simulink library "SHLI_lib"  (Simulink 7.5)
settings: Solver=ode45  StartTime=0.0  StopTime=10.0  RelTol=1e-3
values from neighbouring files (symbols this model uses):
  pSHLI_bool_EparkCheckEnbl = Simulink.Parameter    [SHLI_FAW_par.m]
  pSHLI_bool_EparkStEnbl = Simulink.Parameter    [SHLI_FAW_par.m]
  pSHLI_bool_SBWSafeBtnDisEnbl = Simulink.Parameter    [SHLI_FAW_par.m]
  pSHLI_st_EparkStUnPark = Simulink.Parameter    [SHLI_FAW_par.m]
undefined symbols (not defined in the file or in its folder): EparkModTyp, OperProfTyp, p_bool_False_M, p_bool_True_M, PrkgLockBtnTyp, PrkgLockStsTyp, ShiftLvrPosnTipTyp
libraries: BaseOperationLib_Browser x29, PES_CZ_FAW x3, simulink x1
settings Model: Creator=wuaibin  LastModifiedBy=wuaibin

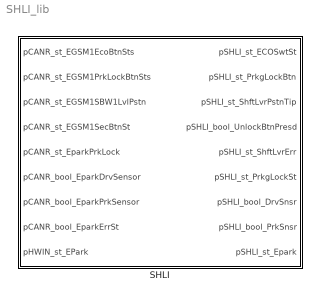
== system SHLI_lib ==
  SHLI : Subsystem  TreatAsAtomicUnit=on

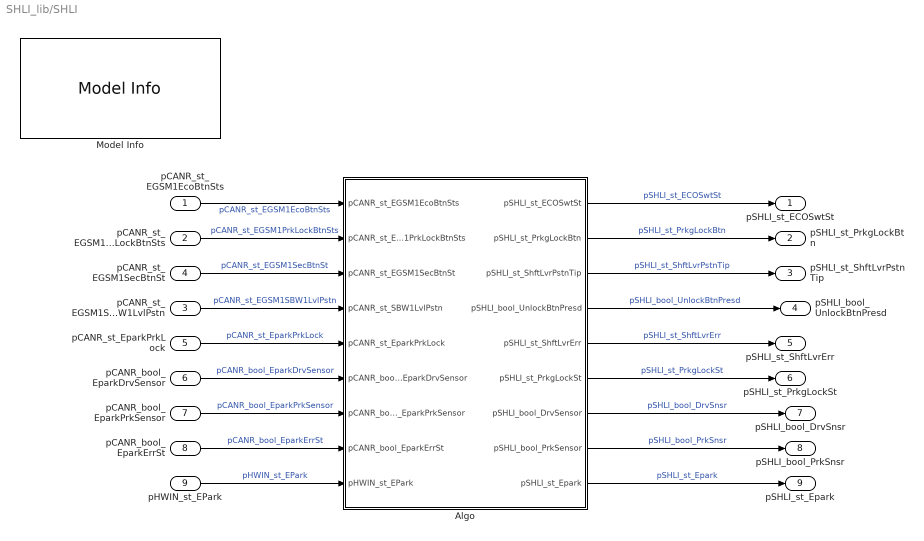
== system SHLI_lib/SHLI ==
  pCANR_st_EGSM1EcoBtnSts : Inport  OutDataType=fixdt(1, 16)  OutScaling=2^0
  pCANR_st_EGSM1PrkLockBtnSts : Inport  Port=2  OutDataType=fixdt(1, 16)  OutScaling=2^0
  pCANR_st_EGSM1SBW1LvlPstn : Inport  Port=3  OutDataType=fixdt(1, 16)  OutScaling=2^0
  pCANR_st_EGSM1SecBtnSt : Inport  Port=4  OutDataType=fixdt(1, 16)  OutScaling=2^0
  pCANR_st_EparkPrkLock : Inport  Port=5  OutDataType=fixdt(1, 16)  OutScaling=2^0
  pCANR_bool_EparkDrvSensor : Inport  Port=6  OutDataType=fixdt(1, 16)  OutScaling=2^0
  pCANR_bool_EparkPrkSensor : Inport  Port=7  OutDataType=fixdt(1, 16)  OutScaling=2^0
  pCANR_bool_EparkErrSt : Inport  Port=8  OutDataType=fixdt(1, 16)  OutScaling=2^0
  pHWIN_st_EPark : Inport  Port=9  OutDataType=fixdt(1, 16)  OutScaling=2^0
  Algo : Subsystem
  Model Info : simulink/Model-Wide Utilities/Model Info  SystemSampleTime=-1  InitialBlockCM=None  BlockCM=None  Frame=on  DisplayStringWithTags=Model Info\nCreated: %<Created>\nCreator: wuaibin  HorizontalTextAlignment=Center  LeftAlignmentValue=0.5  SourceBlockDiagram=HQEV_HCU  TagMaxNumber=20
  pSHLI_st_ECOSwtSt : Outport  OutDataType=fixdt(1, 16)  OutScaling=2^0
  pSHLI_st_PrkgLockBtn : Outport  Port=2  OutDataType=fixdt(1, 16)  OutScaling=2^0
  pSHLI_st_ShftLvrPstnTip : Outport  Port=3  OutDataType=fixdt(1, 16)  OutScaling=2^0
  pSHLI_bool_UnlockBtnPresd : Outport  Port=4  OutDataType=fixdt(1, 16)  OutScaling=2^0
  pSHLI_st_ShftLvrErr : Outport  Port=5  OutDataType=fixdt(1, 16)  OutScaling=2^0
  pSHLI_st_PrkgLockSt : Outport  Port=6  OutDataType=fixdt(1, 16)  OutScaling=2^0
  pSHLI_bool_DrvSnsr : Outport  Port=7  OutDataType=fixdt(1, 16)  OutScaling=2^0
  pSHLI_bool_PrkSnsr : Outport  Port=8  OutDataType=fixdt(1, 16)  OutScaling=2^0
  pSHLI_st_Epark : Outport  Port=9  OutDataType=fixdt(1, 16)  OutScaling=2^0
  wires:
  pCANR_st_EGSM1SBW1LvlPstn/1 -> Algo/4(pCANR_st_SBW1LvlPstn)  "pCANR_st_EGSM1SBW1LvlPstn"
  Algo/2(pSHLI_st_PrkgLockBtn) -> pSHLI_st_PrkgLockBtn/1  "pSHLI_st_PrkgLockBtn"
  Algo/6(pSHLI_st_PrkgLockSt) -> pSHLI_st_PrkgLockSt/1  "pSHLI_st_PrkgLockSt"
  pCANR_st_EGSM1PrkLockBtnSts/1 -> Algo/2(pCANR_st_EGSM1PrkLockBtnSts)  "pCANR_st_EGSM1PrkLockBtnSts"
  Algo/5(pSHLI_st_ShftLvrErr) -> pSHLI_st_ShftLvrErr/1  "pSHLI_st_ShftLvrErr"
  Algo/3(pSHLI_st_ShftLvrPstnTip) -> pSHLI_st_ShftLvrPstnTip/1  "pSHLI_st_ShftLvrPstnTip"
  pCANR_st_EGSM1EcoBtnSts/1 -> Algo/1(pCANR_st_EGSM1EcoBtnSts)  "pCANR_st_EGSM1EcoBtnSts"
  Algo/1(pSHLI_st_ECOSwtSt) -> pSHLI_st_ECOSwtSt/1  "pSHLI_st_ECOSwtSt"
  Algo/8(pSHLI_bool_PrkSensor) -> pSHLI_bool_PrkSnsr/1  "pSHLI_bool_PrkSnsr"
  pCANR_bool_EparkErrSt/1 -> Algo/8(pCANR_bool_EparkErrSt)  "pCANR_bool_EparkErrSt"
  pCANR_bool_EparkDrvSensor/1 -> Algo/6(pCANR_bool_EparkDrvSensor)  "pCANR_bool_EparkDrvSensor"
  pCANR_bool_EparkPrkSensor/1 -> Algo/7(pCANR_bool_EparkPrkSensor)  "pCANR_bool_EparkPrkSensor"
  pCANR_st_EparkPrkLock/1 -> Algo/5(pCANR_st_EparkPrkLock)  "pCANR_st_EparkPrkLock"
  pCANR_st_EGSM1SecBtnSt/1 -> Algo/3(pCANR_st_EGSM1SecBtnSt)  "pCANR_st_EGSM1SecBtnSt"
  pHWIN_st_EPark/1 -> Algo/9(pHWIN_st_EPark)  "pHWIN_st_EPark"
  Algo/9(pSHLI_st_Epark) -> pSHLI_st_Epark/1  "pSHLI_st_Epark"
  Algo/4(pSHLI_bool_UnlockBtnPresd) -> pSHLI_bool_UnlockBtnPresd/1  "pSHLI_bool_UnlockBtnPresd"
  Algo/7(pSHLI_bool_DrvSensor) -> pSHLI_bool_DrvSnsr/1  "pSHLI_bool_DrvSnsr"

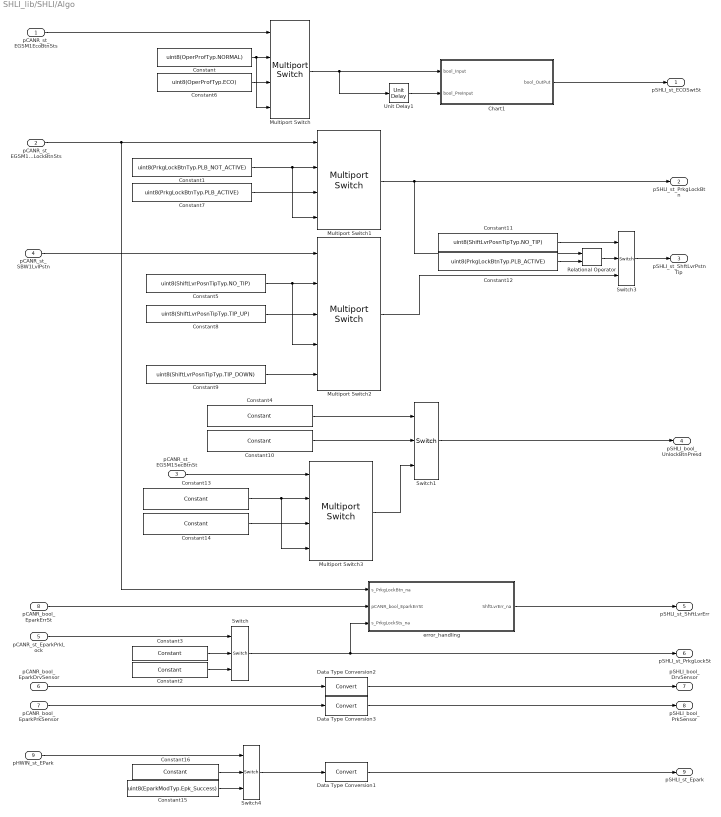
== system SHLI_lib/SHLI/Algo ==
  pCANR_st_EGSM1EcoBtnSts : Inport  OutDataType=fixdt(1, 16)  OutScaling=2^0
  pCANR_st_EGSM1PrkLockBtnSts : Inport  Port=2  OutDataType=fixdt(1, 16)  OutScaling=2^0
  pCANR_st_EGSM1SecBtnSt : Inport  Port=3  OutDataType=fixdt(1, 16)  OutScaling=2^0
  pCANR_st_SBW1LvlPstn : Inport  Port=4  OutDataType=fixdt(1, 16)  OutScaling=2^0
  pCANR_st_EparkPrkLock : Inport  Port=5  OutDataType=fixdt(1, 16)  OutScaling=2^0
  pCANR_bool_EparkDrvSensor : Inport  Port=6  OutDataType=fixdt(1, 16)  OutScaling=2^0
  pCANR_bool_EparkPrkSensor : Inport  Port=7  OutDataType=fixdt(1, 16)  OutScaling=2^0
  pCANR_bool_EparkErrSt : Inport  Port=8  OutDataType=fixdt(1, 16)  OutScaling=2^0
  pHWIN_st_EPark : Inport  Port=9  OutDataType=fixdt(1, 16)  OutScaling=2^0
  Chart1 : Stateflow chart  TreatAsAtomicUnit=on
  Constant : Constant  Value=uint8(OperProfTyp.NORMAL)  OutDataType=fixdt(1, 16)  OutScaling=2^0
      mask Display: patch([0 1 1 1 .75], [1 1 0 .75 1], [0 1 0]);
  Constant1 : Constant  Value=uint8(PrkgLockBtnTyp.PLB_NOT_ACTIVE)  OutDataType=fixdt(1, 16)  OutScaling=2^0
      mask Display: patch([0 1 1 1 .75], [1 1 0 .75 1], [0 1 0]);
  Constant10 : BaseOperationLib_Browser/Sources&Sinks/Constant  Value=pSHLI_bool_SBWSafeBtnDisEnbl  OutMin=[]  OutMax=[]  OutDataType=fixdt(1, 16)  ConRadixGroup=Use specified scaling  OutScaling=2^0  OutDataTypeStr=Inherit: Inherit from 'Constant value'
  Constant11 : Constant  Value=uint8(ShiftLvrPosnTipTyp.NO_TIP)  OutDataType=fixdt(1, 16)  OutScaling=2^0
      mask Display: patch([0 1 1 1 .75], [1 1 0 .75 1], [0 1 0]);
  Constant12 : Constant  Value=uint8(PrkgLockBtnTyp.PLB_ACTIVE)  OutDataType=fixdt(1, 16)  OutScaling=2^0
      mask Display: patch([0 1 1 1 .75], [1 1 0 .75 1], [0 1 0]);
  Constant13 : BaseOperationLib_Browser/Sources&Sinks/Constant  Value=p_bool_False_M  OutMin=[]  OutMax=[]  OutDataType=fixdt(1, 16)  ConRadixGroup=Use specified scaling  OutScaling=2^0  OutDataTypeStr=Inherit: Inherit from 'Constant value'
  Constant14 : BaseOperationLib_Browser/Sources&Sinks/Constant  Value=p_bool_True_M  OutMin=[]  OutMax=[]  OutDataType=fixdt(1, 16)  ConRadixGroup=Use specified scaling  OutScaling=2^0  OutDataTypeStr=Inherit: Inherit from 'Constant value'
  Constant15 : Constant  Value=uint8(EparkModTyp.Epk_Success)  OutDataTypeMode=uint8  OutDataType=fixdt(1, 16)  OutScaling=2^0  OutDataTypeStr=uint8
  Constant16 : BaseOperationLib_Browser/Sources&Sinks/Constant  Value=pSHLI_bool_EparkCheckEnbl  OutMin=[]  OutMax=[]  OutDataType=fixdt(1, 16)  ConRadixGroup=Use specified scaling  OutScaling=2^0  OutDataTypeStr=Inherit: Inherit from 'Constant value'
  Constant2 : BaseOperationLib_Browser/Sources&Sinks/Constant  Value=pSHLI_st_EparkStUnPark  OutMin=[]  OutMax=[]  OutDataType=fixdt(1, 16)  ConRadixGroup=Use specified scaling  OutScaling=2^0  OutDataTypeStr=Inherit: Inherit from 'Constant value'
  Constant3 : BaseOperationLib_Browser/Sources&Sinks/Constant  Value=pSHLI_bool_EparkStEnbl  OutMin=[]  OutMax=[]  OutDataType=fixdt(1, 16)  ConRadixGroup=Use specified scaling  OutScaling=2^0  OutDataTypeStr=Inherit: Inherit from 'Constant value'
  Constant4 : BaseOperationLib_Browser/Sources&Sinks/Constant  Value=p_bool_True_M  OutMin=[]  OutMax=[]  OutDataType=fixdt(1, 16)  ConRadixGroup=Use specified scaling  OutScaling=2^0  OutDataTypeStr=Inherit: Inherit from 'Constant value'
  Constant5 : Constant  Value=uint8(ShiftLvrPosnTipTyp.NO_TIP)  OutDataType=fixdt(1, 16)  OutScaling=2^0
      mask Display: patch([0 1 1 1 .75], [1 1 0 .75 1], [0 1 0]);
  Constant6 : Constant  Value=uint8(OperProfTyp.ECO)  OutDataType=fixdt(1, 16)  OutScaling=2^0
      mask Display: patch([0 1 1 1 .75], [1 1 0 .75 1], [0 1 0]);
  Constant7 : Constant  Value=uint8(PrkgLockBtnTyp.PLB_ACTIVE)  OutDataType=fixdt(1, 16)  OutScaling=2^0
      mask Display: patch([0 1 1 1 .75], [1 1 0 .75 1], [0 1 0]);
  Constant8 : Constant  Value=uint8(ShiftLvrPosnTipTyp.TIP_UP)  OutDataType=fixdt(1, 16)  OutScaling=2^0
      mask Display: patch([0 1 1 1 .75], [1 1 0 .75 1], [0 1 0]);
  Constant9 : Constant  Value=uint8(ShiftLvrPosnTipTyp.TIP_DOWN)  OutDataType=fixdt(1, 16)  OutScaling=2^0
      mask Display: patch([0 1 1 1 .75], [1 1 0 .75 1], [0 1 0]);
  Data Type Conversion1 : DataTypeConversion  OutDataType=fixdt(1, 16)  OutScaling=2^0
  Data Type Conversion2 : DataTypeConversion  OutDataType=fixdt(1, 16)  OutScaling=2^0
  Data Type Conversion3 : DataTypeConversion  OutDataType=fixdt(1, 16)  OutScaling=2^0
  Multiport Switch : BaseOperationLib_Browser/Signal Routing Changed/Multiport Switch  DataPortOrder=Specify indices  Inputs=3  DataPortIndices={uint8(EcoBtnStsTyp.ECO_OFF),uint8(EcoBtnStsTyp.ECO_ON),uint8(EcoBtnStsTyp.ECO_ERROR)}  zeroidx=off  InputSameDT=on  OutMin=[]  OutMax=[]  OutDataType=fixdt(1, 16)  OutScaling=2^0  SaturateOnIntegerOverflow=on
  Multiport Switch1 : BaseOperationLib_Browser/Signal Routing Changed/Multiport Switch  DataPortOrder=Specify indices  Inputs=3  DataPortIndices={uint8(PrkgLockBtnTyp.PLB_NOT_ACTIVE),uint8(PrkgLockBtnTyp.PLB_ACTIVE),uint8(PrkgLockBtnTyp.PLB_ERROR)}  zeroidx=off  InputSameDT=on  OutMin=[]  OutMax=[]  OutDataType=fixdt(1, 16)  OutScaling=2^0  SaturateOnIntegerOverflow=on
  Multiport Switch2 : BaseOperationLib_Browser/Signal Routing Changed/Multiport Switch  DataPortOrder=Specify indices  Inputs=4  DataPortIndices={uint8(FAWShiftLvrPosnTipTyp.FAWTIP_NO_TIP), uint8(FAWShiftLvrPosnTipTyp.FAWTIP_UP), uint8(FAWShiftLvrPosnTipTyp.FAWTIP_DOWN), uint8(FAWShiftLvrPosnTipTyp.FAWTIP_ERROR)}  zeroidx=off  InputSameDT=on  OutMin=[]  OutMax=[]  OutDataType=fixdt(1, 16)  OutScaling=2^0  SaturateOnIntegerOverflow=on
  Multiport Switch3 : BaseOperationLib_Browser/Signal Routing Changed/Multiport Switch  DataPortOrder=Specify indices  Inputs=3  DataPortIndices={uint8(PrkgLockBtnTyp.PLB_NOT_ACTIVE),uint8(PrkgLockBtnTyp.PLB_ACTIVE),uint8(PrkgLockBtnTyp.PLB_ERROR)}  zeroidx=off  InputSameDT=on  OutMin=[]  OutMax=[]  OutDataType=fixdt(1, 16)  OutScaling=2^0  SaturateOnIntegerOverflow=on
  Relational Operator : BaseOperationLib_Browser/Logic Operations Changed/Relational Operator  Operator===  InputSameDT=on  LogicOutDataTypeMode=Specify via dialog  LogicDataType=PDT_Bool  OutDataTypeStr=PDT_Bool
  Switch{,1,3..4} (4 alike) : BaseOperationLib_Browser/Signal Routing Changed/Switch  Criteria=u2 ~= 0  Threshold=1  InputSameDT=on  OutMin=[]  OutMax=[]  OutDataType=fixdt(1,16,0)  OutScaling=[]  SaturateOnIntegerOverflow=on
  Unit Delay1 : BaseOperationLib_Browser/Discrete Unchanged /Unit Delay  X0=0  SampleTime=-1
  error_handling : Subsystem
  pSHLI_st_ECOSwtSt : Outport  OutDataType=fixdt(1, 16)  OutScaling=2^0
  pSHLI_st_PrkgLockBtn : Outport  Port=2  OutDataType=fixdt(1, 16)  OutScaling=2^0
  pSHLI_st_ShftLvrPstnTip : Outport  Port=3  OutDataType=fixdt(1, 16)  OutScaling=2^0
  pSHLI_bool_UnlockBtnPresd : Outport  Port=4  OutDataType=fixdt(1, 16)  OutScaling=2^0
  pSHLI_st_ShftLvrErr : Outport  Port=5  OutDataType=fixdt(1, 16)  OutScaling=2^0
  pSHLI_st_PrkgLockSt : Outport  Port=6  OutDataType=fixdt(1, 16)  OutScaling=2^0
  pSHLI_bool_DrvSensor : Outport  Port=7  OutDataType=fixdt(1, 16)  OutScaling=2^0
  pSHLI_bool_PrkSensor : Outport  Port=8  OutDataType=fixdt(1, 16)  OutScaling=2^0
  pSHLI_st_Epark : Outport  Port=9  OutDataType=fixdt(1, 16)  OutScaling=2^0
  wires:
  pCANR_bool_EparkErrSt/1 -> error_handling/2(pCANR_bool_EparkErrSt)
  error_handling/1(ShftLvrErr_na) -> pSHLI_st_ShftLvrErr/1
  Constant5/1 -> Multiport Switch2/2, Multiport Switch2/4
  Constant/1 -> Multiport Switch/4, Multiport Switch/2
  Constant6/1 -> Multiport Switch/3
  pCANR_st_SBW1LvlPstn/1 -> Multiport Switch2/1
  pCANR_st_EGSM1PrkLockBtnSts/1 -> error_handling/1(s_PrkgLockBtn_na), Multiport Switch1/1
  pCANR_st_EGSM1EcoBtnSts/1 -> Multiport Switch/1
  Constant1/1 -> Multiport Switch1/2, Multiport Switch1/4
  Constant7/1 -> Multiport Switch1/3
  pCANR_st_EparkPrkLock/1 -> Switch/1
  Switch/1 -> error_handling/3(s_PrkgLockSts_na), pSHLI_st_PrkgLockSt/1
  Constant2/1 -> Switch/3
  Constant3/1 -> Switch/2
  pCANR_bool_EparkDrvSensor/1 -> Data Type Conversion2/1
  pCANR_bool_EparkPrkSensor/1 -> Data Type Conversion3/1
  Constant9/1 -> Multiport Switch2/5
  Constant8/1 -> Multiport Switch2/3
  Constant10/1 -> Switch1/2
  Constant4/1 -> Switch1/1
  pCANR_st_EGSM1SecBtnSt/1 -> Multiport Switch3/1
  Switch1/1 -> pSHLI_bool_UnlockBtnPresd/1
  Multiport Switch1/1 -> pSHLI_st_PrkgLockBtn/1, Relational Operator/1
  Chart1/1(bool_OutPut) -> pSHLI_st_ECOSwtSt/1
  Unit Delay1/1 -> Chart1/2(bool_PreInput)
  Multiport Switch/1 -> Chart1/1(bool_Input), Unit Delay1/1
  Constant12/1 -> Relational Operator/2
  Relational Operator/1 -> Switch3/2
  Multiport Switch2/1 -> Switch3/3
  Constant11/1 -> Switch3/1
  Switch3/1 -> pSHLI_st_ShftLvrPstnTip/1
  Data Type Conversion1/1 -> pSHLI_st_Epark/1
  Constant15/1 -> Switch4/3
  Constant16/1 -> Switch4/2
  pHWIN_st_EPark/1 -> Switch4/1
  Switch4/1 -> Data Type Conversion1/1
  Data Type Conversion2/1 -> pSHLI_bool_DrvSensor/1
  Data Type Conversion3/1 -> pSHLI_bool_PrkSensor/1
  Multiport Switch3/1 -> Switch1/3
  Constant13/1 -> Multiport Switch3/2, Multiport Switch3/4
  Constant14/1 -> Multiport Switch3/3

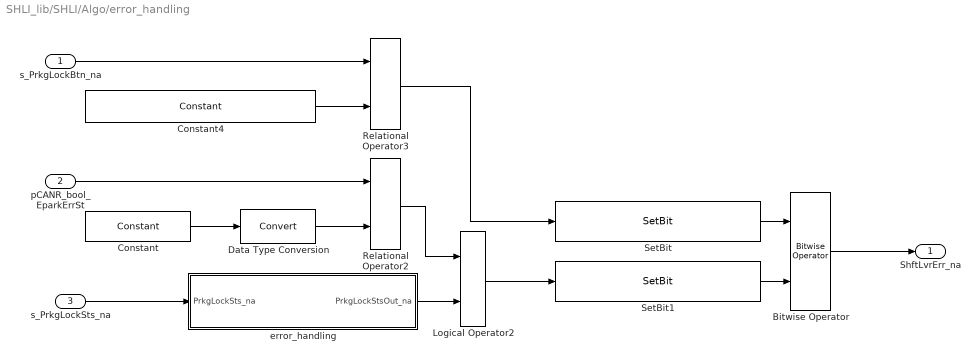
== system SHLI_lib/SHLI/Algo/error_handling ==
  s_PrkgLockBtn_na : Inport  OutDataType=fixdt(1, 16)  OutScaling=2^0
  pCANR_bool_EparkErrSt : Inport  Port=2  OutDataType=fixdt(1, 16)  OutScaling=2^0
  s_PrkgLockSts_na : Inport  Port=3  OutDataType=fixdt(1, 16)  OutScaling=2^0
  Bitwise Operator : BaseOperationLib_Browser/Others Unchanged/Bitwise Operator  logicop=OR  UseBitMask=off  NumInputPorts=2  BitMask=bin2dec('11011001')  BitMaskRealWorld=Stored Integer
  Constant : BaseOperationLib_Browser/Sources&Sinks/Constant  Value=p_bool_True_M  OutMin=[]  OutMax=[]  OutDataType=fixdt(1, 16)  ConRadixGroup=Use specified scaling  OutScaling=2^0  OutDataTypeStr=Inherit: Inherit from 'Constant value'
  Constant4 : BaseOperationLib_Browser/Sources&Sinks/Constant  Value=uint8(PrkgLockBtnTyp.PLB_ERROR)  OutMin=[]  OutMax=[]  OutDataType=Enum: PrkgLockBtnTyp  ConRadixGroup=Best Precision: Vector-wise  OutScaling=[]  OutDataTypeStr=Inherit: Inherit from 'Constant value'
  Data Type Conversion : DataTypeConversion  OutDataType=fixdt(1, 16)  OutScaling=2^0
  Logical Operator2 : BaseOperationLib_Browser/Logic Operations Changed/Logical Operator  Operator=OR  Inputs=2  AllPortsSameDT=on  OutDataTypeMode=Specify via dialog  LogicDataType=PDT_Bool  OutDataTypeStr=PDT_Bool
  Relational Operator2 : BaseOperationLib_Browser/Logic Operations Changed/Relational Operator  Operator===  InputSameDT=on  LogicOutDataTypeMode=Specify via dialog  LogicDataType=PDT_Bool  OutDataTypeStr=PDT_Bool
  Relational Operator3 : BaseOperationLib_Browser/Logic Operations Changed/Relational Operator  Operator===  InputSameDT=on  LogicOutDataTypeMode=Specify via dialog  LogicDataType=PDT_Bool  OutDataTypeStr=PDT_Bool
  SetBit : PES_CZ_FAW/Discontinuities/SetBit  SystemSampleTime=-1  maska=ShftLvrErrTyp.SHIFT_LEVER_ERROR
  SetBit1 : PES_CZ_FAW/Discontinuities/SetBit  SystemSampleTime=-1  maska=ShftLvrErrTyp.E_PARK_ERROR
  error_handling : Subsystem
  ShftLvrErr_na : Outport
  wires:
  Constant4/1 -> Relational Operator3/2
  Constant/1 -> Data Type Conversion/1
  s_PrkgLockBtn_na/1 -> Relational Operator3/1
  pCANR_bool_EparkErrSt/1 -> Relational Operator2/1
  Bitwise Operator/1 -> ShftLvrErr_na/1
  SetBit1/1 -> Bitwise Operator/2
  SetBit/1 -> Bitwise Operator/1
  s_PrkgLockSts_na/1 -> error_handling/1(PrkgLockSts_na)
  Data Type Conversion/1 -> Relational Operator2/2
  Logical Operator2/1 -> SetBit1/1
  Relational Operator3/1 -> SetBit/1
  Relational Operator2/1 -> Logical Operator2/1
  error_handling/1(PrkgLockStsOut_na) -> Logical Operator2/2

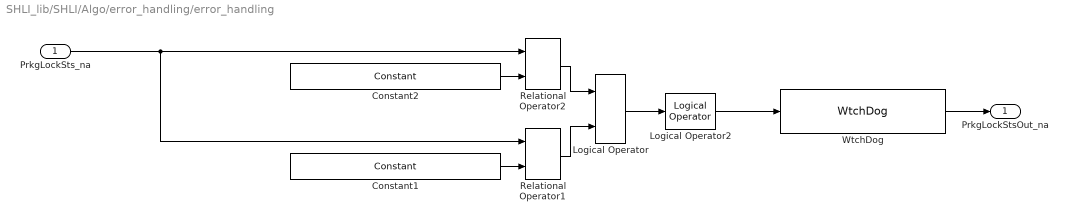
== system SHLI_lib/SHLI/Algo/error_handling/error_handling ==
  PrkgLockSts_na : Inport
  Constant1 : BaseOperationLib_Browser/Sources&Sinks/Constant  Value=uint8(PrkgLockStsTyp.PLS_PARKED)  OutMin=[]  OutMax=[]  OutDataType=Enum: PrkgLockStsTyp  ConRadixGroup=Best Precision: Vector-wise  OutScaling=[]  OutDataTypeStr=Inherit: Inherit from 'Constant value'
  Constant2 : BaseOperationLib_Browser/Sources&Sinks/Constant  Value=uint8(PrkgLockStsTyp.PLS_UNPARKED)  OutMin=[]  OutMax=[]  OutDataType=Enum: PrkgLockStsTyp  ConRadixGroup=Best Precision: Vector-wise  OutScaling=[]  OutDataTypeStr=Inherit: Inherit from 'Constant value'
  Logical Operator : BaseOperationLib_Browser/Logic Operations Changed/Logical Operator  Operator=AND  Inputs=2  AllPortsSameDT=on  OutDataTypeMode=Specify via dialog  LogicDataType=PDT_Bool  OutDataTypeStr=PDT_Bool
  Logical Operator2 : BaseOperationLib_Browser/Logic Operations Changed/Logical Operator  Operator=NOT  Inputs=1  AllPortsSameDT=on  OutDataTypeMode=Specify via dialog  LogicDataType=PDT_Bool  OutDataTypeStr=PDT_Bool
  Relational Operator1 : BaseOperationLib_Browser/Logic Operations Changed/Relational Operator  Operator=~=  InputSameDT=on  LogicOutDataTypeMode=Specify via dialog  LogicDataType=PDT_Bool  OutDataTypeStr=PDT_Bool
  Relational Operator2 : BaseOperationLib_Browser/Logic Operations Changed/Relational Operator  Operator=~=  InputSameDT=on  LogicOutDataTypeMode=Specify via dialog  LogicDataType=PDT_Bool  OutDataTypeStr=PDT_Bool
  WtchDog : PES_CZ_FAW/Discontinuities/WtchDog  SystemSampleTime=-1  timeoutthres=pSHLI_s_TiDlyPrkLock
  PrkgLockStsOut_na : Outport
  wires:
  WtchDog/1 -> PrkgLockStsOut_na/1
  PrkgLockSts_na/1 -> Relational Operator1/1, Relational Operator2/1
  Logical Operator/1 -> Logical Operator2/1
  Relational Operator1/1 -> Logical Operator/2
  Relational Operator2/1 -> Logical Operator/1
  Constant1/1 -> Relational Operator1/2
  Constant2/1 -> Relational Operator2/2
  Logical Operator2/1 -> WtchDog/1

== stateflow chart SHLI/Algo/Chart1 ==
  state Normal
    en:
    bool_OutPut=OperProfTyp.NORMAL;
  state ECO
    en:
    bool_OutPut=OperProfTyp.ECO;
  (default) -> Normal
  Normal -> ECO : [bool_PreInput==OperProfTyp.NORMAL&&...
      | bool_Input==OperProfTyp.ECO]
  ECO -> Normal : [bool_PreInput==OperProfTyp.NORMAL&&...
      | bool_Input==OperProfTyp.ECO]
  data: bool_Input input double; bool_OutPut output uint8; bool_PreInput input double
